simulink library "tire"  (R2020b)
settings: Solver=VariableStepAuto  StartTime=0.0  StopTime=10.0  RelTol=1e-3
undefined symbols (not defined in the file or in its folder): MF_coeff, tire_data
libraries: RF_transformations x6, Resettable_Unit_Delay x4, $bdroot x4, Resettable_Derivative x2, simulink x1, Resettable_Integrator x1
(part 1 of 2)
settings Model: Creator=matte  LastModifiedBy=matteolarcher
settings SFSimCC: CustomCodeUndefinedFunction=UseInterfaceOnly
settings RTWCC: MakeCommand="make_rtw OPTS=\" -D_TS_TYPES_ \""

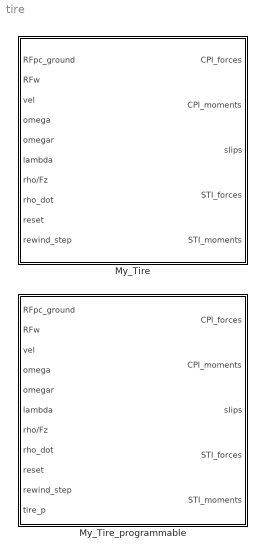
== system tire ==
  My_Tire : Subsystem  TreatAsAtomicUnit=on  SystemSampleTime=Ts_tire  mask{Ts_tire=1e-3, tmp_tire_data=MF_coeff, enabled_rewind_tire=on, PauseResume=0, userSide=2 Right, um=5: Fx,Fy,Mx,My,Mz combined force/moment calculation + turn slip, enabled_transient=on, pressure_from=tire pressure from tir file, tire_p=1, Fz_flag=off}
      mask prompts: Ts_tire "Sampling time"; tmp_tire_data "tire_data"; enabled_rewind_tire "Enable Rewind"; um "Use  mode"; enabled_transient "transient"; pressure_from "Custom tire pressure"; tire_p "Inflation pressure (bar)"; Fz_flag "External Fz"
      mask init:
      | %% self modifications in case of rewind 
      | tire_init_cb(gcb, enabled_rewind_tire, pressure_from);
      | 
      | 
      | % Check tir file side if field exists
      | if isfield(tmp_tire_data, 'TYRESIDE')
      |     if strfind(upper(tmp_tire_data.TYRESIDE),'LEFT')
      |         tirFileSide = 1; % 1 is equal to left
      |     else
      |         tirFileSide = 2; % 2 is equal to right
      |     end
      | else
      |     % Default value
      |     tirFileSide = 2; % 2 is equal to right
      | end
      | 
      | % Create a variable to fip the forces depending on the tire side
      | if isequal(tirFileSide, userSide)
      |     flipSide = 0; % No need to flip the tire, user has specified the same side as in the TIR file
      | else
      |     flipSide = 1; % The user has specified a different tire side from the TIR file
      | end
      | 
      | % Keep only the numeric fields (avoir Simulink errors) and save it into parameterStruct
      | fn = fieldnames(tmp_tire_data);
      | for k = 1:numel(fn)
      |     v = tmp_tire_data.(fn{k});
      |     if(isnumeric(v))
      |         tire_data.(fn{k}) = v;
      |     end
      | end
      | 
      | % set tire pressure 
      | if pressure_from == 1
      |   if tire_data.FITTYP == 52
      |       tire_p = 0;
      |   else 
      |   tire_p = tire_data.INFLPRES;
      |   end 
      | end
      | 
      | % set variable for variant subsystem
      | transient = enabled_transient;
      | 
      | % compute USE_MODE
      | USE_MODE = ((um-1) + 10 * enabled_transient) * (1-2*flipSide);  % um-1 because um is the option number and starts from 1 
      | 
      | % % initialize tire class
      | % TIRE = pacejka_model_62_class(tire_data,USE_MODE);
      settings: RTWFcnNameOpts=Use subsystem name  RTWFileNameOpts=Use subsystem name  FunctionInterfaceSpec=Allow arguments (Optimized)  FunctionWithSeparateData=on
      mask Callback enabled_rewind_tire:
      | A = get_param(gcb,'enabled_rewind_tire');
      | m = Simulink.Mask.get(gcb);
      | 
      | p1 = m.getParameter('PauseResume');
      | 
      | if strcmp(A, 'on')
      |     %set_param(strcat(gcb,'/Transient Slips variant/transient/rewind_variant'),'OverrideUsingVariant','rewind');
      |     p1.Enabled = 'on';
      | %    p1.Visible = 'on';
      | else
      |     %set_param(strcat(gcb,'/Transient Slips variant/transient/rewind_variant'),'OverrideUsingVariant','NO_rewind');
      |     p1.Enabled = 'off';
      | %    p1.Visible = 'off';
      | end
      mask TypeOptions userSide: 1 Left | 2 Right
      mask TypeOptions um: 0: Fz only, no Magic Formula evaluation | 1: Fx,My only | 2: Fy,Mx,Mz only | 3: Fx,Fy,Mx,My,Mz uncombined force/moment calculation | 4: Fx,Fy,Mx,My,Mz combined force/moment calculation | 5: Fx,Fy,Mx,My,Mz combined force/moment calculation + turn slip
      mask TypeOptions pressure_from: tire pressure from tir file | tire pressure from dialog | tire pressure from input port
      mask Callback pressure_from:
      | A = get_param(gcb,'pressure_from');
      | m = Simulink.Mask.get(gcb);
      | p1 = m.getParameter('tire_p');
      | 
      | 
      | if strcmp(A,'tire pressure from dialog')
      |     p1.Enabled = 'on';
      | %    p1.Visible = 'on';
      | else
      |     p1.Enabled = 'off';
      | %    p1.Visible = 'off';
      | end
      mask DialogControl Container3 Prompt: Rewind
      mask DialogControl PauseResume Tooltip: structure with fields rewind_time and rewind_samp
      mask DialogControl Container5 Prompt: Use mode
      mask DialogControl Container4 Prompt: Tire Pressure
      mask DialogControl Fz_flag Tooltip: External vertical force must be connected at the rho/Fz port
  My_Tire_programmable : Subsystem  TreatAsAtomicUnit=on  SystemSampleTime=Ts_tire  mask{Ts_tire=1e-3, tmp_tire_data=MF_coeff, enabled_rewind_tire=on, PauseResume=0, USE_MODE=0, pressure_from=tire pressure from input port, tire_p=1, Fz_flag=0}
      mask prompts: Ts_tire "Sampling time"; tmp_tire_data "tire_data"; enabled_rewind_tire "Enable Rewind"; USE_MODE "Use  mode"; pressure_from "Custom tire pressure"; tire_p "Inflation pressure (Pa)"; Fz_flag "Enable External Fz"
      mask init:
      | %% self modifications in case of rewind 
      | tire_init_cb(gcb, enabled_rewind_tire, pressure_from);
      | 
      | 
      | parsed_um = dec2base(abs(USE_MODE),10) - '0';
      | parsed_um = [zeros(1,2-length(parsed_um)),parsed_um];
      | transient = parsed_um(1);          % transient
      | 
      | 
      | % set tire pressure 
      | if pressure_from == 1
      |   if tire_data.FITTYP == 52
      |       tire_p = 0;
      |   else 
      |   tire_p = tire_data.INFLPRES;
      |   end 
      | end
      | 
      | % Keep only the numeric fields (avoir Simulink errors) and save it into parameterStruct
      | fn = fieldnames(tmp_tire_data);
      | for k = 1:numel(fn)
      |     v = tmp_tire_data.(fn{k});
      |     if(isnumeric(v))
      |         tire_data.(fn{k}) = v;
      |     end
      | end
      | 
      | % % initialize tire class
      | % TIRE = pacejka_model_62_class(tire_data,USE_MODE);
      settings: RTWFcnNameOpts=Use subsystem name  RTWFileNameOpts=Use subsystem name  FunctionInterfaceSpec=Allow arguments (Optimized)  FunctionWithSeparateData=on
      mask Callback enabled_rewind_tire:
      | A = get_param(gcb,'enabled_rewind_tire');
      | m = Simulink.Mask.get(gcb);
      | 
      | p1 = m.getParameter('PauseResume');
      | 
      | if strcmp(A, 'on')
      |     %set_param(strcat(gcb,'/Transient Slips variant/transient/rewind_variant'),'OverrideUsingVariant','rewind');
      |     p1.Enabled = 'on';
      | %    p1.Visible = 'on';
      | else
      |     %set_param(strcat(gcb,'/Transient Slips variant/transient/rewind_variant'),'OverrideUsingVariant','NO_rewind');
      |     p1.Enabled = 'off';
      | %    p1.Visible = 'off';
      | end
      mask TypeOptions pressure_from: tire pressure from tir file | tire pressure from dialog | tire pressure from input port
      mask Callback pressure_from:
      | A = get_param(gcb,'pressure_from');
      | m = Simulink.Mask.get(gcb);
      | p1 = m.getParameter('tire_p');
      | 
      | 
      | if strcmp(A,'tire pressure from dialog')
      |     p1.Enabled = 'on';
      | %    p1.Visible = 'on';
      | else
      |     p1.Enabled = 'off';
      | %    p1.Visible = 'off';
      | end
      mask DialogControl Container3 Prompt: Rewind
      mask DialogControl PauseResume Tooltip: structure with fields rewind_time and rewind_samp
      mask DialogControl Container5 Prompt: Use mode
      mask DialogControl USE_MODE Tooltip: 0: Fz only, no Magic Formula evaluation;<br> 1: Fx,My only;<br> 2: Fy,Mx,Mz only;<br> 3: Fx,Fy,Mx,My,Mz uncombined force/moment calculation;<br> 4: Fx,Fy,Mx,My,Mz combined force/moment calculation;<br> 5: Fx,Fy,Mx,My,Mz combined force/moment calculation + turn slip;<br> +10: transient;<br> *-1: mirroring of tyre characteristics<br>
      mask DialogControl Container4 Prompt: Tire Pressure
      mask DialogControl tire_p Tooltip: Tire pressure [Pa]
      mask DialogControl Fz_flag Tooltip: External vertical force must be connected at the rho/Fz port

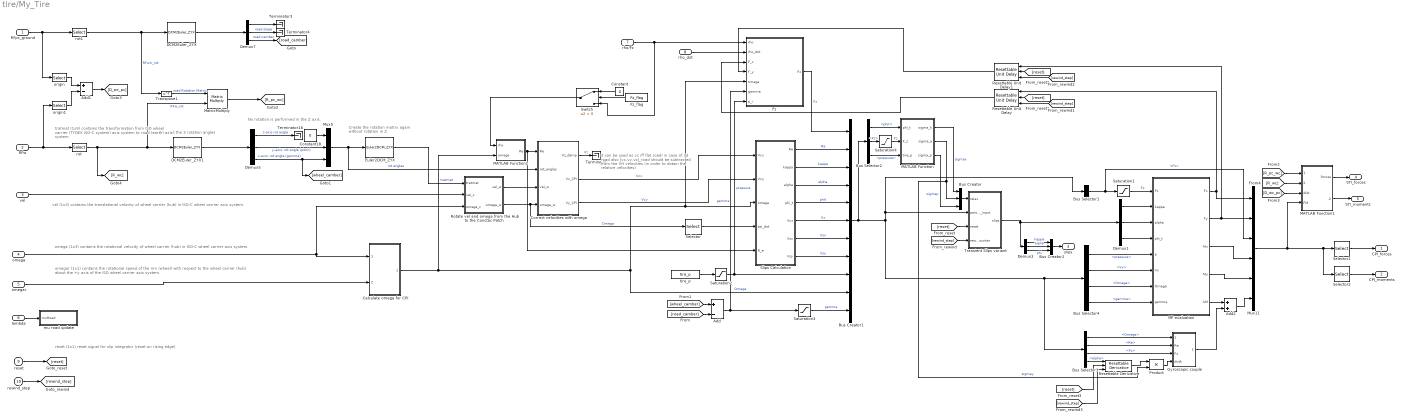
== system tire/My_Tire ==
  note: reset (1x1) reset signal for slip integrator (reset on rising edge)
  note: Get the 3 rotation angles
  note: vel (1x3) contains the translational velocity of wheel carrier (hub) in ISO-C wheel carrier axis system.
  note: Create the rotation matrix again without rotation in Z
  note: omega (1x3) contains the rotational velocity of wheel carrier (hub) in ISO-C wheel carrier axis system.
  note: tratmat (1x9) contains the transformation from ISO wheel carrier (TYDEX ISO-C system) axis system to road (earth) axis system.
  note: omegar (1x1) contains the rotational speed of the rim (wheel) with respect to the wheel carrier (hub) about the +y axis of the ISO wheel carrier axis system.
  note: No rotation is performed in the Z axis.
  note: it can be used as vz iff flat road!
      | in case of 3d road also [vx,vy,vz]_road
      | should be subtracted from the VH velocities
      | (in order to obtain the relative velocities)
  RFpc_ground : Inport
  RFw : Inport  Port=2
  vel : Inport  Port=3
  omega : Inport  Port=4
  omegar : Inport  Port=5
  lambda : Inport  Port=6
  rho/Fz : Inport  Port=7
  rho_dot : Inport  Port=8
  reset : Inport  Port=9
  rewind_step : Inport  Port=10
  Add : Sum  Inputs=+-
  Add1 : Sum  Inputs=+-
  Add2 : Sum
  Bus Creator : BusCreator  Inputs=3
  Bus Creator1 : BusCreator  Inputs=11
  Bus Creator2 : BusCreator  Inputs=3
  Bus Selector1 : BusSelector  OutputSignals=Fz
  Bus Selector2 : BusSelector  OutputSignals=phit,Fz,pressure
  Bus Selector3 : BusSelector  OutputSignals=Omega,Re,Fz,alpha
  Bus Selector4 : BusSelector  OutputSignals=pressure,Vx,Omega,gamma
  Calculate omega for CPI : Subsystem
  Constant : Constant  Value=0
  Constant18 : Constant  Value=0
  Correct velocities with omega : Subsystem
  DCM2Euler_ZYX : RF_transformations/DCM2Euler_ZYX  SystemSampleTime=-1  VariantActivationTime=update diagram  Latency=0  AutoFrameSizeCalculation=off
  DCM2Euler_ZYX1 : RF_transformations/DCM2Euler_ZYX  SystemSampleTime=-1  VariantActivationTime=update diagram  Latency=0  AutoFrameSizeCalculation=off
  Demux{1,3,5,7} (4 alike) : Demux  Outputs=3
  Euler2DCM_ZYX : RF_transformations/Euler2DCM_ZYX  SystemSampleTime=-1  VariantActivationTime=update diagram  Latency=0  AutoFrameSizeCalculation=off
  Fz : MATLAB Function  TreatAsAtomicUnit=on
  Fz_flag : Constant  Value=Fz_flag
  Gyroscopic couple : MATLAB Function  TreatAsAtomicUnit=on
  MATLAB Function : MATLAB Function  TreatAsAtomicUnit=on
  MATLAB Function1 : MATLAB Function  TreatAsAtomicUnit=on
  MATLAB Function2 : MATLAB Function  TreatAsAtomicUnit=on
  MF evaluation : MATLAB Function  TreatAsAtomicUnit=on
  MatrixMultiply : Product  Multiplication=Matrix(*)
  Mux11 : Mux  Inputs=6
  Mux5 : Mux  Inputs=3
  Product : Product
  Resettable Derivative : Resettable_Derivative/Resettable Derivative  Ts_int=Ts_tire  X0_int=0  en_res_flag=enabled_rewind_tire
  Resettable Unit Delay : Resettable_Unit_Delay/Resettable Unit Delay  Ts_int=Ts_tire  X0_int=0  en_res_flag=enabled_rewind_tire
  Resettable Unit Delay1 : Resettable_Unit_Delay/Resettable Unit Delay  Ts_int=Ts_tire  X0_int=0  en_res_flag=enabled_rewind_tire
  Rotate vel and omega from the Hub to the Conctac Patch : Subsystem
  Saturation1 : Saturate  UpperLimit=tire_data.FZMAX  LowerLimit=tire_data.FZMIN
  Saturation2 : Saturate  UpperLimit=tire_data.PRESMAX  LowerLimit=tire_data.PRESMIN  ZeroCross=off
  Saturation3 : Saturate  UpperLimit=tire_data.CAMMAX  LowerLimit=tire_data.CAMMIN
  Saturation4 : Saturate  UpperLimit=tire_data.FZMAX  LowerLimit=tire_data.FZMIN
  Selector : Selector  InputPortWidth=3  IndexOptions=Index vector (dialog)  Indices=[3]  OutputSizes=1
  Selector1 : Selector  InputPortWidth=6  IndexOptions=Index vector (dialog)  Indices=[1:3]  OutputSizes=1
  Selector2 : Selector  InputPortWidth=6  IndexOptions=Index vector (dialog)  Indices=[4:6]  OutputSizes=1
  Slips Calculation : MATLAB Function  TreatAsAtomicUnit=on
  Switch : Switch  Criteria=u2 > Threshold
  Terminator{,3..4,16} (4 alike) : Terminator
  Transient Slips variant : Subsystem  Variant=on
  Transpose1 : Math  Operator=transpose  SignedPower=on  SaturateOnIntegerOverflow=on
  mu road update : MATLAB Function  TreatAsAtomicUnit=on
  origin : Selector  NumberOfDimensions=2  InputPortWidth=3  IndexOptions=Index vector (dialog),Index vector (dialog)  Indices=[1 2 3],[4]  OutputSizes=1,1
  origin1 : Selector  NumberOfDimensions=2  InputPortWidth=3  IndexOptions=Index vector (dialog),Index vector (dialog)  Indices=[1 2 3],[4]  OutputSizes=1,1
  rot : Selector  NumberOfDimensions=2  InputPortWidth=3  IndexOptions=Index vector (dialog),Index vector (dialog)  Indices=[1 2 3],[1 2 3]  OutputSizes=1,1
  rot1 : Selector  NumberOfDimensions=2  InputPortWidth=3  IndexOptions=Index vector (dialog),Index vector (dialog)  Indices=[1 2 3],[1 2 3]  OutputSizes=1,1
  tire_p : Constant  Value=tire_p
  CPI_forces : Outport  VectorParamsAs1DForOutWhenUnconnected=off
  CPI_moments : Outport  Port=2  VectorParamsAs1DForOutWhenUnconnected=off
  slips : Outport  Port=3  VectorParamsAs1DForOutWhenUnconnected=off
  STI_forces : Outport  Port=4
  STI_moments : Outport  Port=5
  wires:
  MATLAB Function/3(sigma_p) -> Bus Creator/3  "sigmap"
  Resettable Unit Delay/1 -> Fz/3(F_x)
  Fz/1(Fz) -> Bus Creator1/1  "Fz"
  [R_wc] -> MATLAB Function1/2(rot_mat_wc)
  Add1/1 -> [D_wc_pc]
  MATLAB Function1/2(moments) -> STI_moments/1
  MATLAB Function1/1(forces) -> STI_forces/1
  Saturation1/1 -> MF evaluation/1(Fz)  "Fz"
  [D_wc_pc] -> MATLAB Function1/3(dist)
  origin1/1 -> Add1/2
  origin/1 -> Add1/1
  [R_pc_wc] -> MATLAB Function1/1(rot_mat_pc_wc)
  MatrixMultiply/1 -> [R_pc_wc]
  Bus Selector2/3 -> MATLAB Function/3(tire_p)  "<pressure>"
  Bus Selector2/2 -> Saturation4/1  "<Fz>"
  Bus Selector2/1 -> MATLAB Function/1(phi_t)  "<phit>"
  Saturation2/1 -> Fz/7(p_i), Bus Creator1/9  "pressure"
  tire_p/1 -> Saturation2/1
  [rewind_step] -> Transient Slips variant/4(rew_counter)
  rewind_step/1 -> [rewind_step]
  [reset] -> Transient Slips variant/3(reset)
  reset/1 -> [reset]
  rho/Fz/1 -> Switch/3, Fz/1(rho)
  Demux3/1 -> Bus Creator2/1  "kappa"
  Demux3/2 -> Bus Creator2/2  "alpha"
  Add/1 -> Fz/6(gamma), Saturation3/1  "gamma"
  [road_camber] -> Add/2
  [wheel_camber] -> Add/1
  rot1/1 -> DCM2Euler_ZYX/1, Transpose1/1  "RFwrr_rot"
  DCM2Euler_ZYX/1 -> Demux7/1
  Transpose1/1 -> MatrixMultiply/1  "road Rotation Matrix"
  Demux7/2 -> Terminator4/1  "road slope"
  Demux7/1 -> Terminator3/1
  Demux7/3 -> [road_camber]  "road camber"
  Correct velocities with omega/1(Vz_damp) -> Terminator/1  "Vz"
  MATLAB Function2/1(Re) -> Correct velocities with omega/1(Re), Slips Calculation/5(R_e)
  Transient Slips variant/1(slips) -> Demux3/1, Demux1/1
  rot/1 -> DCM2Euler_ZYX1/1, MatrixMultiply/2, [R_wc]  "RFw_rot"
  MF evaluation/1(Fx) -> Resettable Unit Delay/1, Mux11/1
  Slips Calculation/5(Vcx) -> Bus Creator1/6  "Vx"
  Slips Calculation/6(Vsx) -> Bus Creator1/7  "Vsx"
  Slips Calculation/2(kappa) -> Bus Creator1/3  "kappa"
  Bus Selector1/1 -> Saturation1/1, Mux11/3  "<Fz>"
  Bus Selector4/2 -> MF evaluation/6(Vx)  "<Vx>"
  Correct velocities with omega/3(Vy_CPI) -> Slips Calculation/2(Vcy)  "Vcy"
  Demux1/2 -> MF evaluation/3(alpha)
  Bus Selector4/3 -> MF evaluation/7(Omega)  "<Omega>"
  Calculate omega for CPI/1(omega_CPI) -> MATLAB Function2/2(omega), Slips Calculation/3(omega), Fz/5(omega), Bus Creator1/10  "Omega"
  Slips Calculation/7(Vsy) -> Bus Creator1/8  "Vsy"
  Bus Creator1/1 -> Bus Selector2/1, Bus Selector1/1, Transient Slips variant/2(parsed_input), Bus Selector3/1, Bus Selector4/1
  Slips Calculation/4(phi_t) -> Bus Creator1/5  "phit"
  Slips Calculation/3(alpha) -> Bus Creator1/4  "alpha"
  Bus Selector4/4 -> MF evaluation/8(gamma)  "<gamma>"
  Slips Calculation/1(Re) -> Bus Creator1/2  "Re"
  Bus Selector4/1 -> MF evaluation/5(p)  "<pressure>"
  Correct velocities with omega/2(Vx_CPI) -> Slips Calculation/1("Vcx ")  "Vcx"
  MF evaluation/2(Fy) -> Resettable Unit Delay1/1, Mux11/2
  MF evaluation/3(Mx) -> Mux11/4
  MF evaluation/4(My) -> Mux11/5
  MF evaluation/5(AM) -> Add2/1
  lambda/1 -> mu road update/1(muRoad)
  MATLAB Function/1(sigma_k) -> Bus Creator/1  "sigmax"
  MATLAB Function/2(sigma_a) -> Bus Creator/2, Product/2  "sigmay"
  Bus Creator/1 -> Transient Slips variant/1(relax)
  Rotate vel and omega from the Hub to the Conctac Patch/1(vel_w) -> Correct velocities with omega/3(vel_w)
  DCM2Euler_ZYX1/1 -> Demux5/1
  Demux5/3 -> Mux5/3, [wheel_camber]  "x-axis: rot angle (gamma)"
  Constant18/1 -> Mux5/1
  Euler2DCM_ZYX/1 -> Rotate vel and omega from the Hub to the Conctac Patch/1(tratmat)  "tratmat"
  omegar/1 -> Calculate omega for CPI/2(omegar)
  Demux5/1 -> Terminator16/1  "z-axis rot angle"
  Mux5/1 -> Euler2DCM_ZYX/1, Correct velocities with omega/2(rot_angles)  "rot angles"
  omega/1 -> Rotate vel and omega from the Hub to the Conctac Patch/3(omega_c), Calculate omega for CPI/1(omega_c)
  RFw/1 -> origin1/1, rot/1
  vel/1 -> Rotate vel and omega from the Hub to the Conctac Patch/2(vel_c)
  Demux5/2 -> Mux5/2  "y-axis: rot angle (pitch)"
  Rotate vel and omega from the Hub to the Conctac Patch/2(omega_w) -> Correct velocities with omega/4(omega_w), Selector/1  "Omega"
  Selector/1 -> Slips Calculation/4(psi_dot)
  Mux11/1 -> MATLAB Function1/4(FM), Selector2/1, Selector1/1
  Demux1/1 -> MF evaluation/2(kappa)
  Demux3/3 -> Bus Creator2/3  "phi"
  Demux1/3 -> MF evaluation/4(phi_t)
  Saturation3/1 -> Bus Creator1/11  "gamma"
  Constant/1 -> Switch/1
  Fz_flag/1 -> Switch/2
  rho_dot/1 -> Fz/2(rho_dot)
  Switch/1 -> MATLAB Function2/1(rho)
  Selector1/1 -> CPI_forces/1
  Selector2/1 -> CPI_moments/1
  RFpc_ground/1 -> origin/1, rot1/1
  Add2/1 -> Mux11/6
  Gyroscopic couple/1(Mz_gyr) -> Add2/2
  Bus Selector3/1 -> Gyroscopic couple/1(Omega)  "<Omega>"
  Bus Selector3/2 -> Gyroscopic couple/2(Re)  "<Re>"
  Bus Selector3/4 -> Resettable Derivative/1  "<alpha>"
  Bus Selector3/3 -> Gyroscopic couple/3(Fz)  "<Fz>"
  Resettable Derivative/1 -> Product/1
  Product/1 -> Gyroscopic couple/4(dvdt)
  [reset] -> Resettable Unit Delay/2
  [rewind_step] -> Resettable Unit Delay/3
  [rewind_step] -> Resettable Unit Delay1/3
  [reset] -> Resettable Unit Delay1/2
  Resettable Unit Delay1/1 -> Fz/4(F_y)
  [reset] -> Resettable Derivative/2
  [rewind_step] -> Resettable Derivative/3
  Bus Creator2/1 -> slips/1
  Saturation4/1 -> MATLAB Function/2(F_z)  "Fz"

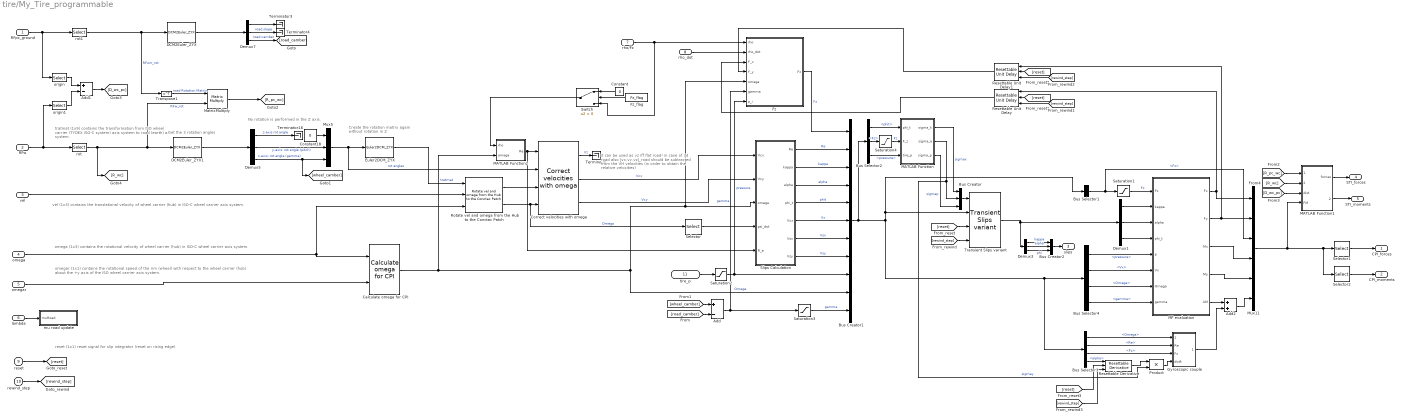
== system tire/My_Tire_programmable ==
  note: it can be used as vz iff flat road!
      | in case of 3d road also [vx,vy,vz]_road
      | should be subtracted from the VH velocities
      | (in order to obtain the relative velocities)
  note: omegar (1x1) contains the rotational speed of the rim (wheel) with respect to the wheel carrier (hub) about the +y axis of the ISO wheel carrier axis system.
  note: tratmat (1x9) contains the transformation from ISO wheel carrier (TYDEX ISO-C system) axis system to road (earth) axis system.
  note: No rotation is performed in the Z axis.
  note: Create the rotation matrix again without rotation in Z
  note: Get the 3 rotation angles
  note: omega (1x3) contains the rotational velocity of wheel carrier (hub) in ISO-C wheel carrier axis system.
  note: vel (1x3) contains the translational velocity of wheel carrier (hub) in ISO-C wheel carrier axis system.
  note: reset (1x1) reset signal for slip integrator (reset on rising edge)
  RFpc_ground : Inport
  RFw : Inport  Port=2
  vel : Inport  Port=3
  omega : Inport  Port=4
  omegar : Inport  Port=5
  lambda : Inport  Port=6
  rho/Fz : Inport  Port=7
  rho_dot : Inport  Port=8
  reset : Inport  Port=9
  rewind_step : Inport  Port=10
  tire_p : Inport  Port=11
  Add : Sum  Inputs=+-
  Add1 : Sum  Inputs=+-
  Add2 : Sum
  Bus Creator : BusCreator  Inputs=3
  Bus Creator1 : BusCreator  Inputs=11
  Bus Creator2 : BusCreator  Inputs=3
  Bus Selector1 : BusSelector  OutputSignals=Fz
  Bus Selector2 : BusSelector  OutputSignals=phit,Fz,pressure
  Bus Selector3 : BusSelector  OutputSignals=Omega,Re,Fz,alpha
  Bus Selector4 : BusSelector  OutputSignals=pressure,Vx,Omega,gamma
  Calculate omega for CPI : $bdroot/My_Tire/Calculate omega for CPI  SystemSampleTime=-1  VariantActivationTime=update diagram  Latency=0  AutoFrameSizeCalculation=off
  Constant : Constant  Value=0
  Constant18 : Constant  Value=0
  Correct velocities with omega : $bdroot/My_Tire/Correct velocities with omega  SystemSampleTime=-1  VariantActivationTime=update diagram  Latency=0  AutoFrameSizeCalculation=off
  DCM2Euler_ZYX : RF_transformations/DCM2Euler_ZYX  SystemSampleTime=-1  VariantActivationTime=update diagram  Latency=0  AutoFrameSizeCalculation=off
  DCM2Euler_ZYX1 : RF_transformations/DCM2Euler_ZYX  SystemSampleTime=-1  VariantActivationTime=update diagram  Latency=0  AutoFrameSizeCalculation=off
  Demux{1,3,5,7} (4 alike) : Demux  Outputs=3
  Euler2DCM_ZYX : RF_transformations/Euler2DCM_ZYX  SystemSampleTime=-1  VariantActivationTime=update diagram  Latency=0  AutoFrameSizeCalculation=off
  Fz : MATLAB Function  TreatAsAtomicUnit=on
  Fz_flag : Constant  Value=Fz_flag
  Gyroscopic couple : MATLAB Function  TreatAsAtomicUnit=on
  MATLAB Function : MATLAB Function  TreatAsAtomicUnit=on
  MATLAB Function1 : MATLAB Function  TreatAsAtomicUnit=on
  MATLAB Function2 : MATLAB Function  TreatAsAtomicUnit=on
  MF evaluation : MATLAB Function  TreatAsAtomicUnit=on
  MatrixMultiply : Product  Multiplication=Matrix(*)
  Mux11 : Mux  Inputs=6
  Mux5 : Mux  Inputs=3
  Product : Product
  Resettable Derivative : Resettable_Derivative/Resettable Derivative  Ts_int=Ts_tire  X0_int=0  en_res_flag=enabled_rewind_tire
  Resettable Unit Delay : Resettable_Unit_Delay/Resettable Unit Delay  Ts_int=Ts_tire  X0_int=0  en_res_flag=enabled_rewind_tire
  Resettable Unit Delay1 : Resettable_Unit_Delay/Resettable Unit Delay  Ts_int=Ts_tire  X0_int=0  en_res_flag=enabled_rewind_tire
  Rotate vel and omega from the Hub to the Conctac Patch : $bdroot/My_Tire/Rotate vel and omega  from the Hub to the Conctac Patch  SystemSampleTime=-1  VariantActivationTime=update diagram  Latency=0  AutoFrameSizeCalculation=off
  Saturation1 : Saturate  UpperLimit=tire_data.FZMAX  LowerLimit=tire_data.FZMIN
  Saturation2 : Saturate  UpperLimit=tire_data.PRESMAX  LowerLimit=tire_data.PRESMIN  ZeroCross=off
  Saturation3 : Saturate  UpperLimit=tire_data.CAMMAX  LowerLimit=tire_data.CAMMIN
  Saturation4 : Saturate  UpperLimit=tire_data.FZMAX  LowerLimit=tire_data.FZMIN
  Selector : Selector  InputPortWidth=3  IndexOptions=Index vector (dialog)  Indices=[3]  OutputSizes=1
  Selector1 : Selector  InputPortWidth=6  IndexOptions=Index vector (dialog)  Indices=[1:3]  OutputSizes=1
  Selector2 : Selector  InputPortWidth=6  IndexOptions=Index vector (dialog)  Indices=[4:6]  OutputSizes=1
  Slips Calculation : MATLAB Function  TreatAsAtomicUnit=on
  Switch : Switch  Criteria=u2 > Threshold
  Terminator{,3..4,16} (4 alike) : Terminator
  Transient Slips variant : $bdroot/My_Tire/Transient Slips variant  SystemSampleTime=-1  VariantActivationTime=update diagram  Latency=0  AutoFrameSizeCalculation=off
  Transpose1 : Math  Operator=transpose  SignedPower=on  SaturateOnIntegerOverflow=on
  mu road update : MATLAB Function  TreatAsAtomicUnit=on
  origin : Selector  NumberOfDimensions=2  InputPortWidth=3  IndexOptions=Index vector (dialog),Index vector (dialog)  Indices=[1 2 3],[4]  OutputSizes=1,1
  origin1 : Selector  NumberOfDimensions=2  InputPortWidth=3  IndexOptions=Index vector (dialog),Index vector (dialog)  Indices=[1 2 3],[4]  OutputSizes=1,1
  rot : Selector  NumberOfDimensions=2  InputPortWidth=3  IndexOptions=Index vector (dialog),Index vector (dialog)  Indices=[1 2 3],[1 2 3]  OutputSizes=1,1
  rot1 : Selector  NumberOfDimensions=2  InputPortWidth=3  IndexOptions=Index vector (dialog),Index vector (dialog)  Indices=[1 2 3],[1 2 3]  OutputSizes=1,1
  CPI_forces : Outport  VectorParamsAs1DForOutWhenUnconnected=off
  CPI_moments : Outport  Port=2  VectorParamsAs1DForOutWhenUnconnected=off
  slips : Outport  Port=3  VectorParamsAs1DForOutWhenUnconnected=off
  STI_forces : Outport  Port=4
  STI_moments : Outport  Port=5
  wires:
  Bus Selector4/4 -> MF evaluation/8(gamma)  "<gamma>"
  Selector2/1 -> CPI_moments/1
  MATLAB Function/1(sigma_k) -> Bus Creator/1  "sigmax"
  Bus Selector3/4 -> Resettable Derivative/1  "<alpha>"
  Bus Creator/1 -> Transient Slips variant/1
  Demux3/2 -> Bus Creator2/2  "alpha"
  Saturation2/1 -> Fz/7(p_i), Bus Creator1/9  "pressure"
  Resettable Unit Delay1/1 -> Fz/4(F_y)
  [wheel_camber] -> Add/1
  Slips Calculation/7(Vsy) -> Bus Creator1/8  "Vsy"
  Constant/1 -> Switch/1
  Bus Creator1/1 -> Bus Selector2/1, Bus Selector1/1, Transient Slips variant/2, Bus Selector3/1, Bus Selector4/1
  Constant18/1 -> Mux5/1
  rho/Fz/1 -> Switch/3, Fz/1(rho)
  Slips Calculation/2(kappa) -> Bus Creator1/3  "kappa"
  Demux1/1 -> MF evaluation/2(kappa)
  omegar/1 -> Calculate omega for CPI/2
  Switch/1 -> MATLAB Function2/1(rho)
  DCM2Euler_ZYX1/1 -> Demux5/1
  Bus Selector3/3 -> Gyroscopic couple/3(Fz)  "<Fz>"
  vel/1 -> Rotate vel and omega from the Hub to the Conctac Patch/2
  rewind_step/1 -> [rewind_step]
  Rotate vel and omega from the Hub to the Conctac Patch/2 -> Correct velocities with omega/4, Selector/1  "Omega"
  Correct velocities with omega/1 -> Terminator/1  "Vz"
  MF evaluation/5(AM) -> Add2/1
  [rewind_step] -> Resettable Unit Delay/3
  Demux5/3 -> Mux5/3, [wheel_camber]  "x-axis: rot angle (gamma)"
  lambda/1 -> mu road update/1(muRoad)
  Bus Selector4/3 -> MF evaluation/7(Omega)  "<Omega>"
  Demux1/2 -> MF evaluation/3(alpha)
  Slips Calculation/1(Re) -> Bus Creator1/2  "Re"
  Demux5/1 -> Terminator16/1  "z-axis rot angle"
  Bus Creator2/1 -> slips/1
  [D_wc_pc] -> MATLAB Function1/3(dist)
  [reset] -> Resettable Unit Delay/2
  Demux3/3 -> Bus Creator2/3  "phi"
  Demux1/3 -> MF evaluation/4(phi_t)
  [R_wc] -> MATLAB Function1/2(rot_mat_wc)
  Product/1 -> Gyroscopic couple/4(dvdt)
  Bus Selector4/1 -> MF evaluation/5(p)  "<pressure>"
  Rotate vel and omega from the Hub to the Conctac Patch/1 -> Correct velocities with omega/3
  Demux3/1 -> Bus Creator2/1  "kappa"
  rho_dot/1 -> Fz/2(rho_dot)
  MF evaluation/1(Fx) -> Resettable Unit Delay/1, Mux11/1
  Euler2DCM_ZYX/1 -> Rotate vel and omega from the Hub to the Conctac Patch/1  "tratmat"
  Bus Selector2/1 -> MATLAB Function/1(phi_t)  "<phit>"
  Mux5/1 -> Euler2DCM_ZYX/1, Correct velocities with omega/2  "rot angles"
  Correct velocities with omega/3 -> Slips Calculation/2(Vcy)  "Vcy"
  tire_p/1 -> Saturation2/1
  Gyroscopic couple/1(Mz_gyr) -> Add2/2
  Selector1/1 -> CPI_forces/1
  MF evaluation/2(Fy) -> Resettable Unit Delay1/1, Mux11/2
  Add/1 -> Fz/6(gamma), Saturation3/1  "gamma"
  Fz_flag/1 -> Switch/2
  MF evaluation/3(Mx) -> Mux11/4
  Add2/1 -> Mux11/6
  RFpc_ground/1 -> origin/1, rot1/1
  Transient Slips variant/1 -> Demux3/1, Demux1/1
  [R_pc_wc] -> MATLAB Function1/1(rot_mat_pc_wc)
  omega/1 -> Rotate vel and omega from the Hub to the Conctac Patch/3, Calculate omega for CPI/1
  Bus Selector3/2 -> Gyroscopic couple/2(Re)  "<Re>"
  Slips Calculation/3(alpha) -> Bus Creator1/4  "alpha"
  Demux7/3 -> [road_camber]  "road camber"
  MF evaluation/4(My) -> Mux11/5
  Demux7/1 -> Terminator3/1
  Selector/1 -> Slips Calculation/4(psi_dot)
  Resettable Unit Delay/1 -> Fz/3(F_x)
  [rewind_step] -> Resettable Unit Delay1/3
  [reset] -> Resettable Unit Delay1/2
  Calculate omega for CPI/1 -> MATLAB Function2/2(omega), Slips Calculation/3(omega), Fz/5(omega), Bus Creator1/10  "Omega"
  Slips Calculation/5(Vcx) -> Bus Creator1/6  "Vx"
  Fz/1(Fz) -> Bus Creator1/1  "Fz"
  RFw/1 -> origin1/1, rot/1
  Saturation3/1 -> Bus Creator1/11  "gamma"
  Resettable Derivative/1 -> Product/1
  Mux11/1 -> MATLAB Function1/4(FM), Selector2/1, Selector1/1
  MatrixMultiply/1 -> [R_pc_wc]
  Correct velocities with omega/2 -> Slips Calculation/1("Vcx ")  "Vcx"
  MATLAB Function1/2(moments) -> STI_moments/1
  Demux5/2 -> Mux5/2  "y-axis: rot angle (pitch)"
  [reset] -> Resettable Derivative/2
  [rewind_step] -> Resettable Derivative/3
  Bus Selector3/1 -> Gyroscopic couple/1(Omega)  "<Omega>"
  MATLAB Function/2(sigma_a) -> Bus Creator/2, Product/2  "sigmay"
  Saturation4/1 -> MATLAB Function/2(F_z)  "Fz"
  Add1/1 -> [D_wc_pc]
  MATLAB Function1/1(forces) -> STI_forces/1
  Saturation1/1 -> MF evaluation/1(Fz)  "Fz"
  origin1/1 -> Add1/2
  origin/1 -> Add1/1
  Bus Selector4/2 -> MF evaluation/6(Vx)  "<Vx>"
  Bus Selector2/3 -> MATLAB Function/3(tire_p)  "<pressure>"
  Demux7/2 -> Terminator4/1  "road slope"
  [rewind_step] -> Transient Slips variant/4
  [reset] -> Transient Slips variant/3
  reset/1 -> [reset]
  rot1/1 -> DCM2Euler_ZYX/1, Transpose1/1  "RFwrr_rot"
  DCM2Euler_ZYX/1 -> Demux7/1
  Transpose1/1 -> MatrixMultiply/1  "road Rotation Matrix"
  Slips Calculation/6(Vsx) -> Bus Creator1/7  "Vsx"
  MATLAB Function2/1(Re) -> Correct velocities with omega/1, Slips Calculation/5(R_e)
  [road_camber] -> Add/2
  rot/1 -> DCM2Euler_ZYX1/1, MatrixMultiply/2, [R_wc]  "RFw_rot"
  Bus Selector1/1 -> Saturation1/1, Mux11/3  "<Fz>"
  MATLAB Function/3(sigma_p) -> Bus Creator/3  "sigmap"
  Bus Selector2/2 -> Saturation4/1  "<Fz>"
  Slips Calculation/4(phi_t) -> Bus Creator1/5  "phit"

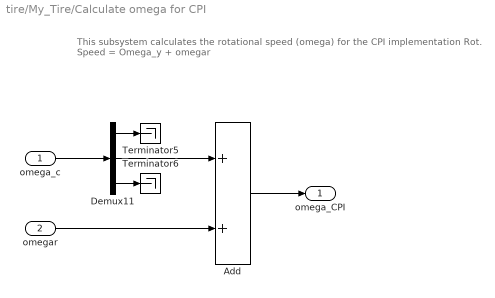
== system tire/My_Tire/Calculate omega for CPI ==
  note: This subsystem calculates the rotational speed (omega) for the CPI implementation
      |
      | Rot. Speed = Omega_y + omegar
  omega_c : Inport
  omegar : Inport  Port=2
  Add : Sum
  Demux11 : Demux  Outputs=3
      settings: DisplayOption=none
  Terminator5 : Terminator
  Terminator6 : Terminator
  omega_CPI : Outport  VectorParamsAs1DForOutWhenUnconnected=off
  wires:
  Demux11/2 -> Add/1
  Demux11/3 -> Terminator6/1
  Demux11/1 -> Terminator5/1
  omegar/1 -> Add/2
  omega_c/1 -> Demux11/1
  Add/1 -> omega_CPI/1

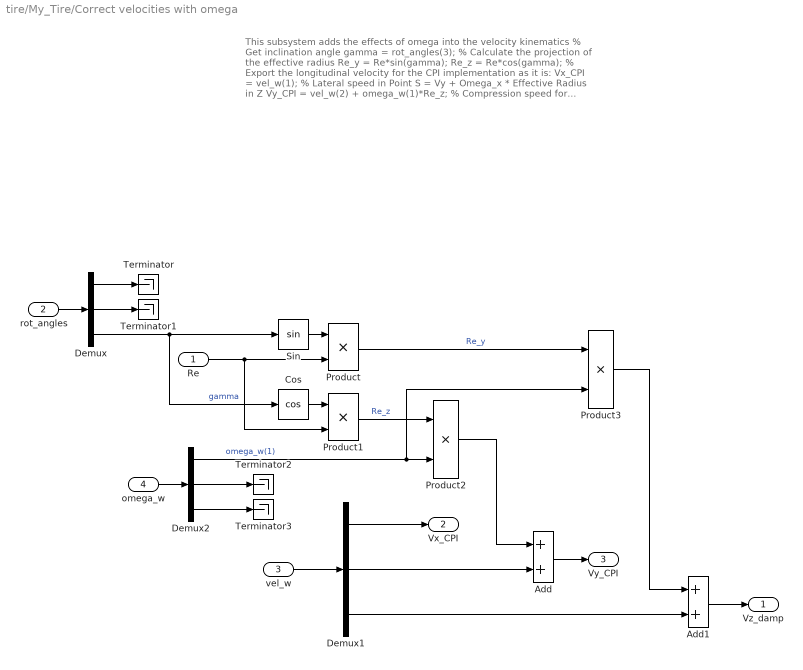
== system tire/My_Tire/Correct velocities with omega ==
  note: This subsystem adds the effects of omega into the velocity kinematics
      |
      | % Get inclination angle
      | gamma = rot_angles(3);
      |
      | % Calculate the projection of the effective radius
      | Re_y = Re*sin(gamma);
      | Re_z = Re*cos(gamma);
      |
      | % Export the longitudinal velocity for the CPI implementation as it is:
      | Vx_CPI = vel_w(1);
      |
      | % Lateral speed in Point S = Vy + Omega_x * Effective Radius in Z
      | Vy_CPI = vel_w(2) + omega_w(1)*Re_z;
      |
      | % Compression speed for damping effects:
      | Vz_damp = vel_w(3) + omega_w(1)*Re_y;
  Re : Inport
  rot_angles : Inport  Port=2
  vel_w : Inport  Port=3
  omega_w : Inport  Port=4
  Add : Sum
  Add1 : Sum
  Cos : Trigonometry  Operator=cos
  Demux : Demux  Outputs=3
      settings: DisplayOption=none
  Demux1 : Demux  Outputs=3
      settings: DisplayOption=none
  Demux2 : Demux  Outputs=3
      settings: DisplayOption=none
  Product{,1..3} (4 alike) : Product
  Sin : Trigonometry
  Terminator{,1..3} (4 alike) : Terminator
  Vz_damp : Outport  VectorParamsAs1DForOutWhenUnconnected=off
  Vx_CPI : Outport  Port=2  VectorParamsAs1DForOutWhenUnconnected=off
  Vy_CPI : Outport  Port=3  VectorParamsAs1DForOutWhenUnconnected=off
  wires:
  rot_angles/1 -> Demux/1
  Demux/1 -> Terminator/1
  Demux/3 -> Sin/1, Cos/1  "gamma"
  Demux/2 -> Terminator1/1
  Sin/1 -> Product/1
  Re/1 -> Product1/2, Product/2
  Cos/1 -> Product1/1
  Product/1 -> Product3/1  "Re_y"
  Product1/1 -> Product2/1  "Re_z"
  vel_w/1 -> Demux1/1
  Demux1/1 -> Vx_CPI/1
  Demux1/2 -> Add/2
  omega_w/1 -> Demux2/1
  Demux2/3 -> Terminator3/1
  Demux2/2 -> Terminator2/1
  Demux2/1 -> Product3/2, Product2/2  "omega_w(1)"
  Product2/1 -> Add/1
  Add/1 -> Vy_CPI/1
  Product3/1 -> Add1/1
  Demux1/3 -> Add1/2
  Add1/1 -> Vz_damp/1

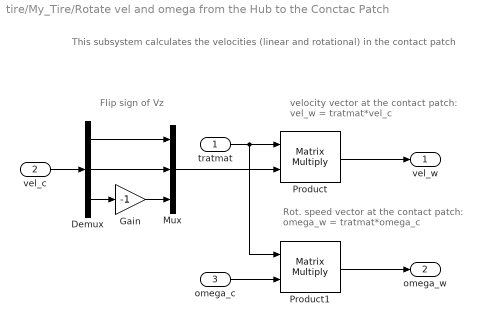
== system tire/My_Tire/Rotate vel and omega from the Hub to the Conctac Patch ==
  note: This subsystem calculates the velocities (linear and rotational) in the contact patch
  note: velocity vector at the contact patch:
      | vel_w = tratmat*vel_c
  note: Flip sign of Vz
  note: Rot. speed vector at the contact patch:
      | omega_w = tratmat*omega_c
  tratmat : Inport
  vel_c : Inport  Port=2
  omega_c : Inport  Port=3
  Demux : Demux  Outputs=3
      settings: DisplayOption=none
  Gain : Gain  Gain=-1
  Mux : Mux  Inputs=3
  Product : Product  Multiplication=Matrix(*)
  Product1 : Product  Multiplication=Matrix(*)
  vel_w : Outport  VectorParamsAs1DForOutWhenUnconnected=off
  omega_w : Outport  Port=2  VectorParamsAs1DForOutWhenUnconnected=off
  wires:
  Gain/1 -> Mux/3
  Product1/1 -> omega_w/1
  omega_c/1 -> Product1/2
  Product/1 -> vel_w/1
  tratmat/1 -> Product/1, Product1/1
  Mux/1 -> Product/2
  Demux/2 -> Mux/2
  Demux/3 -> Gain/1
  Demux/1 -> Mux/1
  vel_c/1 -> Demux/1

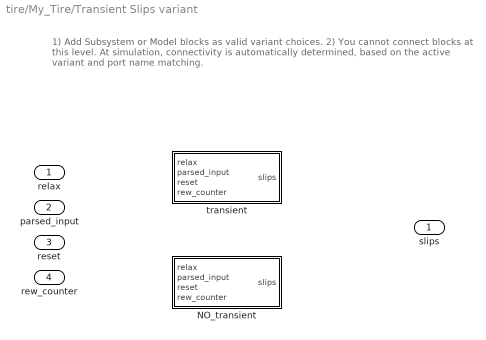
== system tire/My_Tire/Transient Slips variant ==
  note: 1) Add Subsystem or Model blocks as valid variant choices.
      | 2) You cannot connect blocks at this level. At simulation, connectivity is automatically
      | determined, based on the active variant and port name matching.
  relax : Inport
  parsed_input : Inport  Port=2
  reset : Inport  Port=3
  rew_counter : Inport  Port=4
  NO_transient : Subsystem  VariantControl=transient == 0
  transient : Subsystem  VariantControl=transient == 1
  slips : Outport

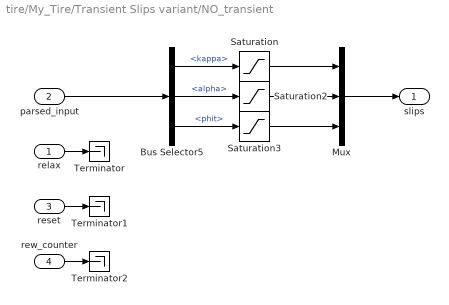
== system tire/My_Tire/Transient Slips variant/NO_transient ==
  relax : Inport
  parsed_input : Inport  Port=2
  reset : Inport  Port=3
  rew_counter : Inport  Port=4
  Bus Selector5 : BusSelector  OutputSignals=kappa,alpha,phit
  Mux : Mux  Inputs=3
  Saturation : Saturate  UpperLimit=tire_data.KPUMAX  LowerLimit=tire_data.KPUMIN
  Saturation2 : Saturate  UpperLimit=tire_data.ALPMAX  LowerLimit=tire_data.ALPMIN
  Saturation3 : Saturate  UpperLimit=10  LowerLimit=-10
  Terminator : Terminator
  Terminator1 : Terminator
  Terminator2 : Terminator
  slips : Outport
  wires:
  Mux/1 -> slips/1
  parsed_input/1 -> Bus Selector5/1
  relax/1 -> Terminator/1
  reset/1 -> Terminator1/1
  rew_counter/1 -> Terminator2/1
  Bus Selector5/1 -> Saturation/1  "<kappa>"
  Bus Selector5/2 -> Saturation2/1  "<alpha>"
  Bus Selector5/3 -> Saturation3/1  "<phit>"
  Saturation/1 -> Mux/1
  Saturation2/1 -> Mux/2
  Saturation3/1 -> Mux/3

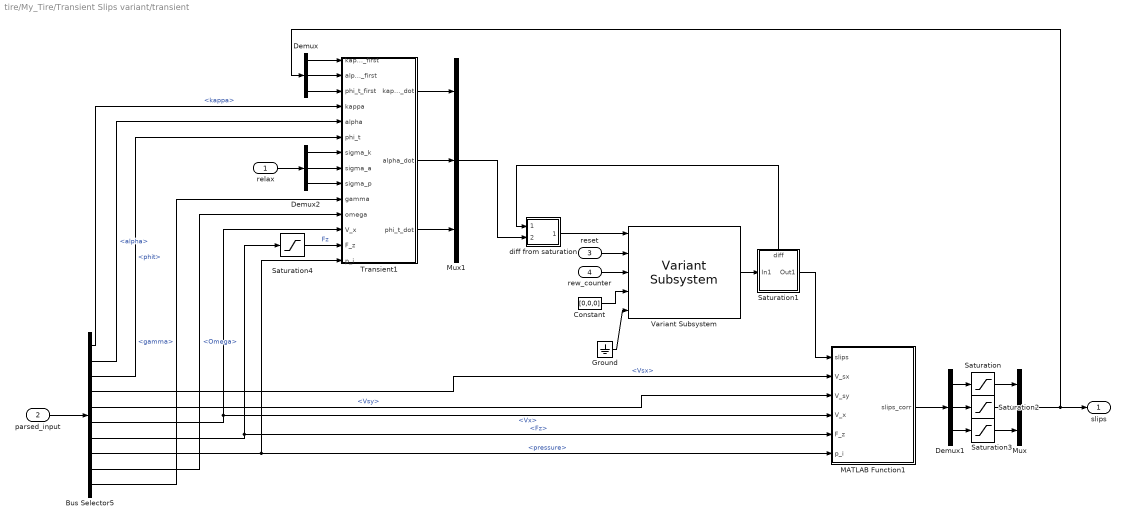
== system tire/My_Tire/Transient Slips variant/transient ==
  relax : Inport
  parsed_input : Inport  Port=2
  reset : Inport  Port=3
  rew_counter : Inport  Port=4
  Bus Selector5 : BusSelector  OutputSignals=kappa,alpha,phit,Vsx,Vsy,Vx,Fz,pressure,Omega,gamma
  Constant : Constant  Value=[0,0,0]
  Demux : Demux  Outputs=3
  Demux1 : Demux  Outputs=3
  Demux2 : Demux  Outputs=3
  Ground : Ground
  MATLAB Function1 : MATLAB Function  TreatAsAtomicUnit=on
  Mux : Mux  Inputs=3
  Mux1 : Mux  Inputs=3
  Saturation : Saturate  UpperLimit=tire_data.KPUMAX  LowerLimit=tire_data.KPUMIN
  Saturation1 : Subsystem
      settings: PortSchema="{\"entries\":[{\"content\":{\"sides\":[{\"content\":{\"connectorIds\":[\"In1\"]},\"type\":\"ConnectorPlacement.EquallySpacedRectSide\",\"uuid\":\"92fa975d-9a01-4e23-b2ef-bf2f52c25c94\"},{\"content\":{\"connectorIds\":[\"Out1\"],\"side\":\"RIGHT\"},\"type\":\"ConnectorPlacement.EquallySpacedRectSide\",\"uuid\":\"148f7a62-c4c2-4d15-85dd-6eaa33fbfd8b\"},{\"content\":{\"connectorIds\":[\"Out2\"],\"side\":\"TOP\"},\"type\":\"ConnectorPlacement.EquallySpacedRectSide\",\"uuid\":\"fd0971a6-b9e7-41a1-933a-0e20c7f9727d\"},{\"content\":{\"connectorIds\":[],\"side\":\"HIDDEN\"},\"type\":\"ConnectorPlacement.EquallySpacedRectSide\",\"uuid\":\"6b9ed3af-9418-4062-a229-79477a07262d\"}]},\"type\":\"ConnectorPlacement.EquallySpacedConnector\",\"uuid\":\"43b5fd82-0743-43b4-91af-ab803132cca7\"}],\"packageUris\":[\"http://schema.mathworks.com/mf0/Connector/R2020b\"],\"version\":\"1.0\"}"
  Saturation2 : Saturate  UpperLimit=tire_data.ALPMAX  LowerLimit=tire_data.ALPMIN
  Saturation3 : Saturate  UpperLimit=10  LowerLimit=-10
  Saturation4 : Saturate  UpperLimit=tire_data.FZMAX  LowerLimit=tire_data.FZMIN
  Transient1 : MATLAB Function  TreatAsAtomicUnit=on
  Variant Subsystem : Resettable_Integrator/Variant Subsystem  Ts_int=Ts_tire  L_up=[inf inf inf]  L_low=[-inf -inf -inf]  en_res_flag=enabled_rewind_tire
  diff from saturation : Subsystem
  slips : Outport
  wires:
  Demux2/3 -> Transient1/9(sigma_p)
  Demux/3 -> Transient1/3(phi_t_first)
  Bus Selector5/6 -> MATLAB Function1/4(V_x), Transient1/12(V_x)  "<Vx>"
  Bus Selector5/3 -> Transient1/6(phi_t)  "<phit>"
  relax/1 -> Demux2/1
  Demux/2 -> Transient1/2(alpha_first)
  Mux/1 -> Demux/1, slips/1
  Bus Selector5/8 -> MATLAB Function1/6(p_i), Transient1/14(p_i)  "<pressure>"
  parsed_input/1 -> Bus Selector5/1
  Demux2/2 -> Transient1/8(sigma_a)
  Bus Selector5/2 -> Transient1/5(alpha)  "<alpha>"
  Transient1/1(kappa_dot) -> Mux1/1
  Saturation1/1(Out1) -> MATLAB Function1/1(slips)
  MATLAB Function1/1(slips_corr) -> Demux1/1
  rew_counter/1 -> Variant Subsystem/3
  Bus Selector5/4 -> MATLAB Function1/2(V_sx)  "<Vsx>"
  Bus Selector5/1 -> Transient1/4(kappa)  "<kappa>"
  Transient1/2(alpha_dot) -> Mux1/2
  Demux/1 -> Transient1/1(kappa_first)
  Bus Selector5/9 -> Transient1/11(omega)  "<Omega>"
  Bus Selector5/5 -> MATLAB Function1/3(V_sy)  "<Vsy>"
  Bus Selector5/7 -> MATLAB Function1/5(F_z), Saturation4/1  "<Fz>"
  Bus Selector5/10 -> Transient1/10(gamma)  "<gamma>"
  Demux2/1 -> Transient1/7(sigma_k)
  Transient1/3(phi_t_dot) -> Mux1/3
  Mux1/1 -> diff from saturation/2(In1)
  Ground/1 -> Variant Subsystem/5
  reset/1 -> Variant Subsystem/2
  Constant/1 -> Variant Subsystem/4
  Saturation4/1 -> Transient1/13(F_z)  "Fz"
  Variant Subsystem/1 -> Saturation1/1(In1)
  Saturation1/2(diff) -> diff from saturation/1(diff)
  diff from saturation/1(Out1) -> Variant Subsystem/1
  Demux1/1 -> Saturation/1
  Saturation/1 -> Mux/1
  Demux1/3 -> Saturation3/1
  Saturation3/1 -> Mux/3
  Saturation2/1 -> Mux/2
  Demux1/2 -> Saturation2/1

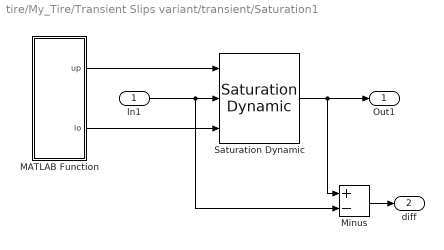
== system tire/My_Tire/Transient Slips variant/transient/Saturation1 ==
  In1 : Inport
  MATLAB Function : MATLAB Function  TreatAsAtomicUnit=on
  Minus : Sum  Inputs=+-
  Saturation Dynamic : simulink/Discontinuities/Saturation Dynamic  OutMin=[]  OutMax=[]  OutDataTypeStr=Inherit: Same as second input  OutDataType=fixdt(1, 16)  OutScaling=2^-10  DoSatur=off
  Out1 : Outport
  diff : Outport  Port=2
  wires:
  Minus/1 -> diff/1
  Saturation Dynamic/1 -> Out1/1, Minus/1
  In1/1 -> Saturation Dynamic/2, Minus/2
  MATLAB Function/2(lo) -> Saturation Dynamic/3
  MATLAB Function/1(up) -> Saturation Dynamic/1

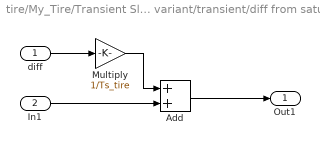
== system tire/My_Tire/Transient Slips variant/transient/diff from saturation ==
  diff : Inport
  In1 : Inport  Port=2
  Add : Sum
  Multiply : Gain  Gain=1/Ts_tire
  Out1 : Outport
  wires:
  Multiply/1 -> Add/1
  In1/1 -> Add/2
  Add/1 -> Out1/1
  diff/1 -> Multiply/1

== matlab function tire/My_Tire_programmable/MATLAB Function1 ==
  data: rot_mat_pc_wc input; rot_mat_wc input; dist input; forces output; FM input; moments output
function [forces, moments] = fcn(rot_mat_pc_wc,rot_mat_wc, dist, FM)


% Rotation of forces and moments:
forces = rot_mat_pc_wc'*FM(1:3);
moments = rot_mat_pc_wc'*FM(4:6) + cross(rot_mat_wc'*dist,forces);

== matlab function tire/My_Tire/MATLAB Function ==
  data: phi_t input; sigma_k output; F_z input; tire_p input; sigma_a output; tire_data parameter; USE_MODE parameter; sigma_p output
function [sigma_k, sigma_a, sigma_p] = calcRelax(phi_t, F_z, tire_p, tire_data, USE_MODE)

% initialize tire class !!! TEMPORARY WORKAROUND !!! 
if tire_data.FITTYP == 62
    TIRE = pacejka_model_62_class(tire_data, USE_MODE);
    [sigma_k, sigma_a, sigma_p] = TIRE.compute_relax( phi_t, F_z, tire_p);
elseif tire_data.FITTYP == 52
    TIRE = pacejka_model_52_class(tire_data, USE_MODE);
    [sigma_k, sigma_a, sigma_p] = TIRE.compute_relax( phi_t, F_z, tire_p);
else
    sigma_k = NaN;
    sigma_a = NaN;
    sigma_p = NaN;
end

== matlab function tire/My_Tire/MATLAB Function1 ==
  data: rot_mat_pc_wc input; rot_mat_wc input; dist input; forces output; FM input; moments output
function [forces, moments] = fcn(rot_mat_pc_wc,rot_mat_wc, dist, FM)


% Rotation of forces and moments:
forces = rot_mat_pc_wc'*FM(1:3);
moments = rot_mat_pc_wc'*FM(4:6) + cross(rot_mat_wc'*dist,forces);

== matlab function tire/My_Tire/MF evaluation ==
  data: Fz input; Fx output; kappa input; alpha input; phi_t input; p input; Vx input; Omega input; gamma input; Fy output; Mx output; My output; AM output; tire_data parameter; USE_MODE parameter
function [Fx,Fy,Mx,My,AM] = fcn(Fz,kappa,alpha,phi_t,p,Vx,Omega,gamma, tire_data, USE_MODE)

% % initialize tire class !!! TEMPORARY WORKAROUND !!! 
if tire_data.FITTYP == 62
    TIRE = pacejka_model_62_class(tire_data, USE_MODE);
    [Fx,Fy,Mx,My,AM] = TIRE.compute_forces(Fz,kappa,alpha,phi_t,Vx,Omega,gamma,p,tire_data);
    %[Fx,Fy,Mx,My,AM] = TIRE.compute_forces(Fz,kappa,alpha,phi_t,Vx,Omega,gamma,p);
elseif tire_data.FITTYP == 52
    TIRE = pacejka_model_52_class(tire_data, USE_MODE);
    [Fx,Fy,Mx,My,AM] = TIRE.compute_forces(Fz,kappa,alpha,phi_t,Vx,Omega,gamma,p,tire_data);
%     %[Fx,Fy,Mx,My,AM] = TIRE.compute_forces(Fz,kappa,alpha,phi_t,Vx,Omega,gamma,p);
else
    Fx = NaN;
    Fy = NaN;
    Mx = NaN;
    My = NaN;
    AM = NaN;
end

end

== matlab function tire/My_Tire/Slips Calculation ==
  data: Re output; kappa output; Vcx input; Vcy input; omega input; alpha output; phi_t output; Vcx output; Vsx output; Vsy output; psi_dot input; R_e input; tire_data parameter; USE_MODE parameter
function [Re, kappa, alpha,phi_t, Vcx, Vsx, Vsy] = calcSlips(Vcx, Vcy, omega, psi_dot, R_e, tire_data, USE_MODE)

% initialize tire class !!! TEMPORARY WORKAROUND !!! 
if tire_data.FITTYP == 62
    TIRE = pacejka_model_62_class(tire_data, USE_MODE);
    [kappa, alpha, phi_t, Vsx, Vsy, Re] = TIRE.compute_slips(Vcx, Vcy, omega, psi_dot, R_e);
elseif tire_data.FITTYP == 52
    TIRE = pacejka_model_52_class(tire_data, USE_MODE);
    [kappa, alpha, phi_t, Vsx, Vsy, Re] = TIRE.compute_slips(Vcx, Vcy, omega, psi_dot, R_e);
else
     kappa = NaN; 
     alpha = NaN;
     phi_t = NaN;
     Vsx = NaN;
     Vsy = NaN;
     Re = NaN;
end

== matlab function tire/My_Tire/Transient Slips variant/transient/MATLAB Function1 ==
  data: slips input; slips_corr output; V_sx input; V_sy input; V_x input; F_z input; p_i input; tire_data parameter; USE_MODE parameter
function slips_corr = fcn(slips, V_sx, V_sy, V_x, F_z, p_i, tire_data, USE_MODE)

% initialize tire class !!! TEMPORARY WORKAROUND !!! 
if tire_data.FITTYP == 62
    TIRE = pacejka_model_62_class(tire_data, USE_MODE);
    [kappa_corr, alpha_corr, phi_t_corr] = TIRE.compute_corrected_slips(slips(1), slips(2), slips(3), V_x, V_sx, V_sy, F_z, p_i);
elseif tire_data.FITTYP == 52
    TIRE = pacejka_model_52_class(tire_data, USE_MODE);
    [kappa_corr, alpha_corr, phi_t_corr] = TIRE.compute_corrected_slips(slips(1), slips(2), slips(3), V_x, V_sx, V_sy, F_z, p_i);
else
    kappa_corr = NaN;
    alpha_corr = NaN;
    phi_t_corr = NaN;
end

slips_corr = [kappa_corr;alpha_corr;phi_t_corr];

end

== matlab function tire/My_Tire/Transient Slips variant/transient/Transient1 ==
  data: kappa_first input; alpha_first input; phi_t_first input; kappa input; kappa_dot output; alpha input; phi_t input; sigma_k input; sigma_a input; sigma_p input; gamma input; omega input; V_x input; F_z input; p_i input; tire_data parameter; alpha_dot output; USE_MODE parameter; phi_t_dot output
function [kappa_dot, alpha_dot, phi_t_dot] = slipsDyn(kappa_first, alpha_first, phi_t_first, kappa, alpha, phi_t, sigma_k, sigma_a, sigma_p, gamma, omega, V_x, F_z, p_i, tire_data, USE_MODE)

% initialize tire class !!! TEMPORARY WORKAROUND !!! 
if tire_data.FITTYP == 62
    TIRE = pacejka_model_62_class(tire_data, USE_MODE);
    [kappa_dot, alpha_dot, phi_t_dot] = TIRE.compute_slips_dot(kappa_first, alpha_first, phi_t_first, kappa, alpha, phi_t, sigma_k, sigma_a, sigma_p, gamma, omega, V_x, F_z, p_i);
elseif tire_data.FITTYP == 52
    TIRE = pacejka_model_52_class(tire_data, USE_MODE);
    [kappa_dot, alpha_dot, phi_t_dot] = TIRE.compute_slips_dot(kappa_first, alpha_first, phi_t_first, kappa, alpha, phi_t, sigma_k, sigma_a, sigma_p, gamma, omega, V_x, F_z, p_i);
else
    kappa_dot = NaN;
    alpha_dot = NaN;
    phi_t_dot = NaN;
end

== matlab function tire/My_Tire_programmable/MATLAB Function2 ==
  data: rho input; omega input; Re output; tire_data parameter; USE_MODE parameter
function Re = fcn(rho, omega,tire_data, USE_MODE)
% initialize tire class !!! TEMPORARY WORKAROUND !!! 
if tire_data.FITTYP == 62
    TIRE = pacejka_model_62_class(tire_data, USE_MODE);
    [Re] = TIRE.compute_Re(rho, omega);
elseif tire_data.FITTYP == 52
    TIRE = pacejka_model_52_class(tire_data, USE_MODE);
    [Re] = TIRE.compute_Re(rho, omega);
else
    Re = NaN;
end

== matlab function tire/My_Tire/mu road update ==
  data: muRoad input; tire_data parameter
function  fcn(muRoad, tire_data)


% Update mux and muy with muRoad
tire_data.LMUX = tire_data.LMUX*muRoad;
tire_data.LMUY = tire_data.LMUY*muRoad;

== matlab function tire/My_Tire_programmable/MF evaluation ==
  data: Fz input; Fx output; kappa input; alpha input; phi_t input; p input; Vx input; Omega input; gamma input; Fy output; Mx output; My output; AM output; tire_data parameter; USE_MODE parameter
function [Fx,Fy,Mx,My,AM] = fcn(Fz,kappa,alpha,phi_t,p,Vx,Omega,gamma, tire_data, USE_MODE)

% % initialize tire class !!! TEMPORARY WORKAROUND !!! 
if tire_data.FITTYP == 62
    TIRE = pacejka_model_62_class(tire_data, USE_MODE);
    [Fx,Fy,Mx,My,AM] = TIRE.compute_forces(Fz,kappa,alpha,phi_t,Vx,Omega,gamma,p,tire_data);
    %[Fx,Fy,Mx,My,AM] = TIRE.compute_forces(Fz,kappa,alpha,phi_t,Vx,Omega,gamma,p);
elseif tire_data.FITTYP == 52
    TIRE = pacejka_model_52_class(tire_data, USE_MODE);
    [Fx,Fy,Mx,My,AM] = TIRE.compute_forces(Fz,kappa,alpha,phi_t,Vx,Omega,gamma,p,tire_data);
%     %[Fx,Fy,Mx,My,AM] = TIRE.compute_forces(Fz,kappa,alpha,phi_t,Vx,Omega,gamma,p);
else
    Fx = NaN;
    Fy = NaN;
    Mx = NaN;
    My = NaN;
    AM = NaN;
end

end

== matlab function tire/My_Tire_programmable/Slips Calculation ==
  data: Re output; kappa output; Vcx input; Vcy input; omega input; alpha output; phi_t output; Vcx output; Vsx output; Vsy output; psi_dot input; R_e input; tire_data parameter; USE_MODE parameter
function [Re, kappa, alpha,phi_t, Vcx, Vsx, Vsy] = calcSlips(Vcx, Vcy, omega, psi_dot, R_e, tire_data, USE_MODE)

% initialize tire class !!! TEMPORARY WORKAROUND !!! 
if tire_data.FITTYP == 62
    TIRE = pacejka_model_62_class(tire_data, USE_MODE);
    [kappa, alpha, phi_t, Vsx, Vsy, Re] = TIRE.compute_slips(Vcx, Vcy, omega, psi_dot, R_e);
elseif tire_data.FITTYP == 52
    TIRE = pacejka_model_52_class(tire_data, USE_MODE);
    [kappa, alpha, phi_t, Vsx, Vsy, Re] = TIRE.compute_slips(Vcx, Vcy, omega, psi_dot, R_e);
else
     kappa = NaN; 
     alpha = NaN;
     phi_t = NaN;
     Vsx = NaN;
     Vsy = NaN;
     Re = NaN;
end

== matlab function tire/My_Tire_programmable/mu road update ==
  data: muRoad input; tire_data parameter
function  fcn(muRoad, tire_data)


% Update mux and muy with muRoad
tire_data.LMUX = tire_data.LMUX*muRoad;
tire_data.LMUY = tire_data.LMUY*muRoad;

== matlab function tire/My_Tire/Gyroscopic couple ==
  data: Omega input; Mz_gyr output; Re input; Fz input; dvdt input; tire_data parameter; USE_MODE parameter
function Mz_gyr = fcn(Omega, Re, Fz, dvdt, tire_data, USE_MODE)

% Mz due to the gyroscopic effect of the yre belt deflections (7.2.5 Book)

parsed_um = dec2base(abs(USE_MODE),10) - '0';
parsed_um = [zeros(1,2-length(parsed_um)),parsed_um];
USE_MODE_1    = parsed_um(2);          % type of calculation

if USE_MODE_1 == 2 || USE_MODE_1 == 3 || USE_MODE_1 == 4 || USE_MODE_1 == 5  
    c_gyr = 0.5; % for a radial ply steel-belted car tire,
    m_t = tire_data.BELT_MASS;
    Fz_0 = tire_data.FNOMIN;
    
    Mz_gyr = c_gyr * m_t * Re * Omega * dvdt * Fz/Fz_0 ;
else
    Mz_gyr = 0;
end

== matlab function tire/My_Tire/Transient Slips variant/transient/Saturation1/MATLAB Function ==
  data: up output; lo output; tire_data parameter
function [up, lo] = fcn(tire_data)

%% Bounds Computation

up = [tire_data.KPUMAX tire_data.ALPMAX 10] ;
lo = [tire_data.KPUMIN tire_data.ALPMIN -10] ;

== matlab function tire/My_Tire/MATLAB Function2 ==
  data: rho input; omega input; Re output; tire_data parameter; USE_MODE parameter
function Re = fcn(rho, omega,tire_data, USE_MODE)
% initialize tire class !!! TEMPORARY WORKAROUND !!! 
if tire_data.FITTYP == 62
    TIRE = pacejka_model_62_class(tire_data, USE_MODE);
    [Re] = TIRE.compute_Re(rho, omega);
elseif tire_data.FITTYP == 52
    TIRE = pacejka_model_52_class(tire_data, USE_MODE);
    [Re] = TIRE.compute_Re(rho, omega);
else
    Re = NaN;
end

== matlab function tire/My_Tire_programmable/Fz ==
  data: rho input; rho_dot input; F_x input; F_y input; omega input; gamma input; p_i input; Fz output; tire_data parameter; USE_MODE parameter; Fz_flag parameter
function Fz = fcn(rho,rho_dot,F_x,F_y,omega,gamma,p_i,tire_data, USE_MODE, Fz_flag)

% !! rho take the value of external Fz in case of Fz_flag ~= 0

if Fz_flag == 0
    % initialize tire class !!! TEMPORARY WORKAROUND !!!
    if tire_data.FITTYP == 62
        TIRE = pacejka_model_62_class(tire_data, USE_MODE);
        Fz = TIRE.compute_F_z(rho, rho_dot, omega, gamma, p_i, F_x, F_y);
    elseif tire_data.FITTYP == 52
        TIRE = pacejka_model_52_class(tire_data, USE_MODE);
        Fz = TIRE.compute_F_z(rho, rho_dot, omega, gamma, p_i, F_x, F_y);
    else
        Fz = NaN;
    end
    
else
    Fz = rho; % Fz passtrough
end
end
